simulink model "s0326"  (Simulink 6.0)
settings: Solver=ode3  SolverMode=SingleTasking  StartTime=0.0  StopTime=900  FixedStep=1  MaxStep=1  RelTol=1e-3  AbsTol=1e-6
values from neighbouring files (symbols this model uses):
  PT1nen = G.den{1}    [m0326.m]
  PT1zae = G.num{1}    [m0326.m]
  Tt = .4    (= 0.4)    [m0108d.m]    (also in m0259.m = 1; m0314.m = 2.13; m0322.m = 0.8; m0326.m = 4)
undefined symbols (not defined in the file or in its folder): Ttnen, Ttzae
settings Model: LastModifiedBy=Froriep
settings DataIOCC: LimitDataPoints=off  SaveOutput=off  SaveTime=off
settings OptimizationCC: BooleanDataType=off
settings DebuggingCC: SolverPrmCheckMsg=none
settings HardwareCC: TargetUnknown=on
settings GRTTargetCC: ModelReferenceCompliant=off  MatFileLogging=off

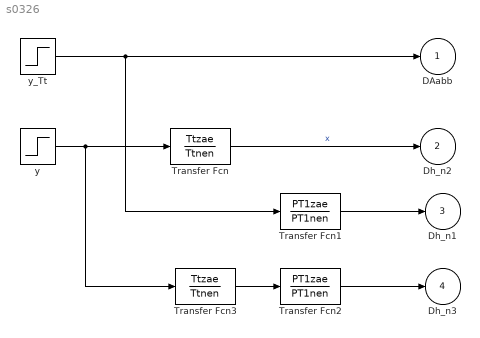
== system s0326 ==
  Transfer Fcn : TransferFcn  Numerator=Ttzae  Denominator=Ttnen
  Transfer Fcn1 : TransferFcn  Numerator=PT1zae  Denominator=PT1nen
  Transfer Fcn2 : TransferFcn  Numerator=PT1zae  Denominator=PT1nen
  Transfer Fcn3 : TransferFcn  Numerator=Ttzae  Denominator=Ttnen
  y : Step  Time=0  SampleTime=0
  y_Tt : Step  Time=Tt  SampleTime=0
  DAabb : Outport
  Dh_n2 : Outport  Port=2
  Dh_n1 : Outport  Port=3
  Dh_n3 : Outport  Port=4
  wires:
  Transfer Fcn/1 -> Dh_n2/1  "x"
  Transfer Fcn1/1 -> Dh_n1/1
  Transfer Fcn3/1 -> Transfer Fcn2/1
  Transfer Fcn2/1 -> Dh_n3/1
  y_Tt/1 -> DAabb/1, Transfer Fcn1/1
  y/1 -> Transfer Fcn/1, Transfer Fcn3/1
